simulink model "PMSM_Simulation"  (R2023a)
settings: Solver=ode23t  StartTime=0.0  StopTime=5  MaxStep=0.2  RelTol=1e-4  EnableMultiTasking=on
InitFcn:
  | p = 4;
  | Ld = 0.000425;
  | Lq = 0.00085;
  | psim = 0.119489;
  | Rs = 0.0485;
  | J = 0.00027;
  | Kpwm = 1;
  | Tsi = 0.0001;
  | h = 900;
  | 
  | L0 = (Ld+Lq)/2;
  | SMO_Kp = 100;
  | SMO_Coef =0.0001;
  | Ki_id = Ld*(h+1)/(4.5*Kpwm*(Tsi^2)*(h^2));
  | Kp_id = Ld*(h+1)/(4.5*Kpwm*Tsi*h);
  | 
  | wc =3000;
  | 
  | Ki_iq = Lq*(h+1)/(4.5*Kpwm*Tsi^2*h^2);
  | Kp_iq = Lq*(h+1)/(4.5*Kpwm*Tsi*h);
  | 
  | 
  | Kp_Spd = pi*J/(300*p*psim*Tsi)
  | Ki_Spd = pi*J/(6000*p*psim*Tsi^2)
  | 
  | DeadTime = 2e-6;
  | 
  | Udc = 650;
model workspace (MAT data in the model file):
  KfDeadCompen_CpPeriodTimesT_NULL : Simulink.Parameter (value not decoded)
  KfMDCC_InvParkCpPeriodTimesT_NULL : Simulink.Parameter (value not decoded)
values from neighbouring files (symbols this model uses):
  KfDeadCompen_SetDeltaTime_us = myPackage.Parameter    [DeadCompen.m]
  VbDeadComp_SwtUseIsttrDes_flg = myPackage.Parameter    [DeadCompen.m]
  VfDeadCompen_agIPredAdpr_C = myPackage.Parameter    [DeadCompen.m]
  VfDeadCompen_ISttrDdeThdSwt_A = myPackage.Parameter    [DeadCompen.m]
  VfDeadCompen_ISttrIgbtThdSwt_A = myPackage.Parameter    [DeadCompen.m]
  VfDeadCompen_rDdeISttrHi_R = myPackage.Parameter    [DeadCompen.m]
  VfDeadCompen_rDdeISttrLo_R = myPackage.Parameter    [DeadCompen.m]
  VfDeadCompen_rIgbtISttrHi_R = myPackage.Parameter    [DeadCompen.m]
  VfDeadCompen_rIgbtISttrLo_R = myPackage.Parameter    [DeadCompen.m]
  VfDeadCompen_uDdeISttrHi_V = myPackage.Parameter    [DeadCompen.m]
  VfDeadCompen_uDdeISttrLo_V = myPackage.Parameter    [DeadCompen.m]
  VfDeadCompen_uIgbtISttrHi_V = myPackage.Parameter    [DeadCompen.m]
  VfDeadCompen_uIgbtISttrLo_V = myPackage.Parameter    [DeadCompen.m]
symbols that are objects in the model workspace (value not decoded): KfDeadCompen_CpPeriodTimesT_NULL, KfMDCC_InvParkCpPeriodTimesT_NULL
undefined symbols (not defined in the file or in its folder): DiscIntNeverNeededParam, TableDeadTime_us, TableDeadTimeLookUpCur_A, VuDeadCompen_agIPredAdpr_C
libraries: simulink x23, mcbcontrolslib x11, mcbplantlib x1, spsCurrentMeasurementLib x1, spsDCVoltageSourceLib x1, spsMultimeterLib x1, spsPermanentMagnetSynchronousMachineLib x1, eePmsmCurrentController x1, spsThreePhaseVIMeasurementLib x1, spsUniversalBridgeLib x1, spspowerguiLib x1
(part 2 of 4)

== system PMSM_Simulation/Subsystem/Subsystem/Subsystem2/Subsystem ==
  U_Phase_Dyc : Inport
  V_Phase_Dyc : Inport  Port=2
  W_Phase_Dyc : Inport  Port=3
  iPhase_U : Inport  Port=4
  iPhase_V : Inport  Port=5
  iPhase_W : Inport  Port=6
  uDcLink : Inport  Port=7
  PwmFreq_Hz : Inport  Port=8
  Bus Creator : BusCreator  Inputs=4
  Bus Creator1 : BusCreator  Inputs=3
  DeadTimeDuty_Calc : Subsystem
  DeltaTimeOnOffDuty_Calc : Subsystem
  DutyErr_Calc : Subsystem  Commented=on  TreatAsAtomicUnit=on
  Tavon_Calc : Subsystem
  Bus_DutyCompensate : Outport
  wires:
  U_Phase_Dyc/1 -> Tavon_Calc/1(U_Phase_Dyc), Bus Creator1/1  "DutyPhaseU"
  V_Phase_Dyc/1 -> Bus Creator1/2, Tavon_Calc/2(V_Phase_Dyc)  "DutyPhaseV"
  W_Phase_Dyc/1 -> Bus Creator1/3, Tavon_Calc/3(W_Phase_Dyc)  "DutyPhaseW"
  iPhase_U/1 -> DeltaTimeOnOffDuty_Calc/1(iPhase_U), Tavon_Calc/4(iPhase_U)
  iPhase_V/1 -> DeltaTimeOnOffDuty_Calc/2(iPhase_V), Tavon_Calc/5(iPhase_V)
  iPhase_W/1 -> DeltaTimeOnOffDuty_Calc/3(iPhase_W), Tavon_Calc/6(iPhase_W)
  uDcLink/1 -> Tavon_Calc/7(uDcLink)
  PwmFreq_Hz/1 -> DeadTimeDuty_Calc/1(PwmFreq_Hz), DeltaTimeOnOffDuty_Calc/4(PwmFreq_Hz)
  Tavon_Calc/1(Bus_DutyAvon) -> Bus Creator/2  "Bus_DutyAvon"
  DeltaTimeOnOffDuty_Calc/1(Bus_DeltaTimeOnOffDuty) -> Bus Creator/3  "Bus_DeltaTimeOnOffDuty"
  DeadTimeDuty_Calc/1(DeadTimeDuty_NULL) -> Bus Creator/4  "DeadTimeDuty_NULL"
  Bus Creator/1 -> Bus_DutyCompensate/1  "Bus_DutyCompensate"
  Bus Creator1/1 -> Bus Creator/1  "SVM_DutyPhase"

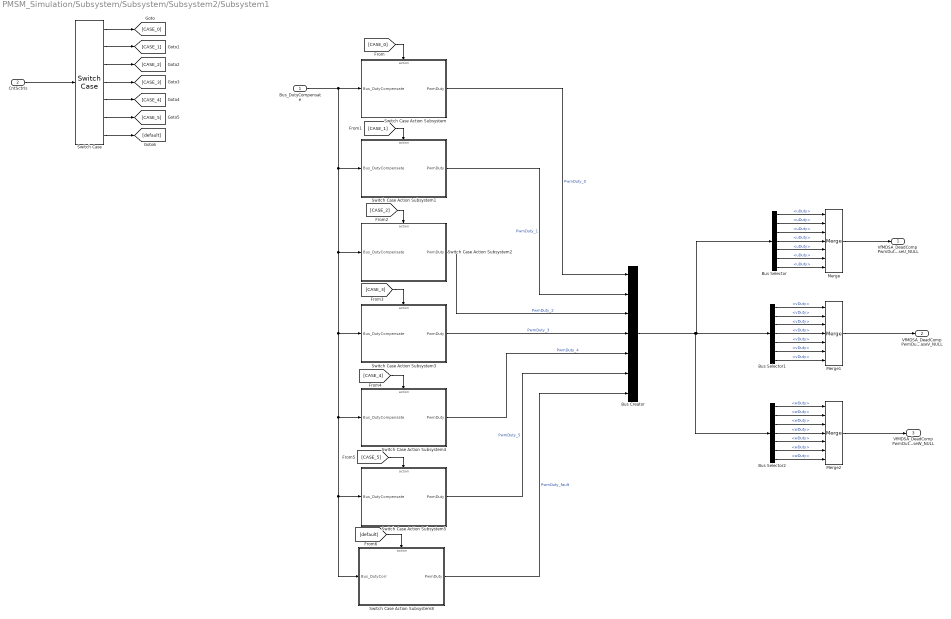
== system PMSM_Simulation/Subsystem/Subsystem/Subsystem2/Subsystem1 ==
  Bus_DutyCompensate : Inport
  CntSctrIs : Inport  Port=2
  Bus Creator : BusCreator  Inputs=7
  Bus Selector : BusSelector  OutputSignals=PwmDuty_0.uDuty,PwmDuty_1.uDuty,PwmDuty_2.uDuty,PwmDuty_3.uDuty,PwmDuty_4.uDuty,PwmDuty_5.uDuty,PwmDuty_fault.uDuty
  Bus Selector1 : BusSelector  OutputSignals=PwmDuty_1.vDuty,PwmDuty_0.vDuty,PwmDuty_2.vDuty,PwmDuty_3.vDuty,PwmDuty_4.vDuty,PwmDuty_5.vDuty,PwmDuty_fault.vDuty
  Bus Selector2 : BusSelector  OutputSignals=PwmDuty_0.wDuty,PwmDuty_1.wDuty,PwmDuty_2.wDuty,PwmDuty_3.wDuty,PwmDuty_4.wDuty,PwmDuty_5.wDuty,PwmDuty_fault.wDuty
  Merge : Merge  Inputs=7
  Merge1 : Merge  Inputs=7
  Merge2 : Merge  Inputs=7
  Switch Case : SwitchCase  CaseConditions={0,1,2,3,4,5}
  Switch Case Action Subsystem : Subsystem  TreatAsAtomicUnit=on
  Switch Case Action Subsystem1 : Subsystem  TreatAsAtomicUnit=on
  Switch Case Action Subsystem2 : Subsystem  TreatAsAtomicUnit=on
  Switch Case Action Subsystem3 : Subsystem  TreatAsAtomicUnit=on
  Switch Case Action Subsystem4 : Subsystem  TreatAsAtomicUnit=on
  Switch Case Action Subsystem5 : Subsystem  TreatAsAtomicUnit=on
  Switch Case Action Subsystem8 : Subsystem  TreatAsAtomicUnit=on
  VfMDSA_DeadCompPwmDutyCyclePhaseU_NULL : Outport
  VfMDSA_DeadCompPwmDutyCyclePhaseV_NULL : Outport  Port=2
  VfMDSA_DeadCompPwmDutyCyclePhaseW_NULL : Outport  Port=3
  wires:
  CntSctrIs/1 -> Switch Case/1
  Switch Case/1 -> [CASE_0]
  Switch Case/2 -> [CASE_1]
  Switch Case/3 -> [CASE_2]
  Switch Case/4 -> [CASE_3]
  Switch Case/5 -> [CASE_4]
  Switch Case/7 -> [default]
  [CASE_0] -> Switch Case Action Subsystem/Action
  [CASE_1] -> Switch Case Action Subsystem1/Action
  [CASE_2] -> Switch Case Action Subsystem2/Action
  [CASE_3] -> Switch Case Action Subsystem3/Action
  [CASE_4] -> Switch Case Action Subsystem4/Action
  [CASE_5] -> Switch Case Action Subsystem5/Action
  [default] -> Switch Case Action Subsystem8/Action
  Switch Case/6 -> [CASE_5]
  Merge/1 -> VfMDSA_DeadCompPwmDutyCyclePhaseU_NULL/1
  Switch Case Action Subsystem/1(PwmDuty) -> Bus Creator/1  "PwmDuty_0"
  Switch Case Action Subsystem1/1(PwmDuty) -> Bus Creator/2  "PwmDuty_1"
  Switch Case Action Subsystem2/1(PwmDuty) -> Bus Creator/3  "PwmDuty_2"
  Switch Case Action Subsystem3/1(PwmDuty) -> Bus Creator/4  "PwmDuty_3"
  Switch Case Action Subsystem4/1(PwmDuty) -> Bus Creator/5  "PwmDuty_4"
  Switch Case Action Subsystem5/1(PwmDuty) -> Bus Creator/6  "PwmDuty_5"
  Switch Case Action Subsystem8/1(PwmDuty) -> Bus Creator/7  "PwmDuty_fault"
  Merge1/1 -> VfMDSA_DeadCompPwmDutyCyclePhaseV_NULL/1
  Merge2/1 -> VfMDSA_DeadCompPwmDutyCyclePhaseW_NULL/1
  Bus Creator/1 -> Bus Selector2/1, Bus Selector1/1, Bus Selector/1
  Bus Selector/1 -> Merge/1  "<uDuty>"
  Bus Selector/2 -> Merge/2  "<uDuty>"
  Bus Selector/3 -> Merge/3  "<uDuty>"
  Bus Selector/4 -> Merge/4  "<uDuty>"
  Bus Selector/5 -> Merge/5  "<uDuty>"
  Bus Selector/6 -> Merge/6  "<uDuty>"
  Bus Selector/7 -> Merge/7  "<uDuty>"
  Bus Selector1/1 -> Merge1/1  "<vDuty>"
  Bus Selector1/2 -> Merge1/2  "<vDuty>"
  Bus Selector1/3 -> Merge1/3  "<vDuty>"
  Bus Selector1/4 -> Merge1/4  "<vDuty>"
  Bus Selector1/5 -> Merge1/5  "<vDuty>"
  Bus Selector1/6 -> Merge1/6  "<vDuty>"
  Bus Selector1/7 -> Merge1/7  "<vDuty>"
  Bus Selector2/1 -> Merge2/1  "<wDuty>"
  Bus Selector2/2 -> Merge2/2  "<wDuty>"
  Bus Selector2/3 -> Merge2/3  "<wDuty>"
  Bus Selector2/4 -> Merge2/4  "<wDuty>"
  Bus Selector2/5 -> Merge2/5  "<wDuty>"
  Bus Selector2/6 -> Merge2/6  "<wDuty>"
  Bus Selector2/7 -> Merge2/7  "<wDuty>"
  Bus_DutyCompensate/1 -> Switch Case Action Subsystem1/1(Bus_DutyCompensate), Switch Case Action Subsystem2/1(Bus_DutyCompensate), Switch Case Action Subsystem3/1(Bus_DutyCompensate), Switch Case Action Subsystem4/1(Bus_DutyCompensate), Switch Case Action Subsystem5/1(Bus_DutyCompensate), Switch Case Action Subsystem8/1("Bus_DutyCorr "), Switch Case Action Subsystem/1(Bus_DutyCompensate)

== system PMSM_Simulation/Subsystem/Subsystem/Subsystem2/Subsystem2 ==
  IsdDes_A : Inport
  IsqDes_A : Inport  Port=2
  IsdFb_A : Inport  Port=3
  IsqFb_A : Inport  Port=4
  FrqRtrEl_Hz : Inport  Port=5
  agPreRtrEl : Inport  Port=6
  PwmFreq_Hz : Inport  Port=7
  Gain : Gain  Gain=6*pi
  Inverse Clarke Transform : mcbcontrolslib/Inverse Clarke Transform
  Inverse Park Transform : mcbcontrolslib/Inverse Park Transform  AxisAlignment=D-axis
  Sine-Cosine Lookup : mcbcontrolslib/Sine-Cosine Lookup  AngleInput=Radians  N_points=4095
  Subsystem1 : Subsystem
  Subsystem3 : Subsystem
  iaPre : Outport
  ibPre : Outport  Port=2
  icPre : Outport  Port=3
  CntSctrIs : Outport  Port=4
  wires:
  Inverse Park Transform/1 -> Inverse Clarke Transform/1
  Subsystem1/2(Isq_A) -> Subsystem3/5(Isq_A), Inverse Park Transform/2
  IsdDes_A/1 -> Subsystem1/1(IsdDes_A)
  Subsystem1/1(Isd_A) -> Inverse Park Transform/1, Subsystem3/4(Isd_A)
  Sine-Cosine Lookup/2 -> Inverse Park Transform/4
  Inverse Clarke Transform/2 -> ibPre/1
  Sine-Cosine Lookup/1 -> Inverse Park Transform/3
  IsqFb_A/1 -> Subsystem1/4(IsqFb_A)
  Inverse Clarke Transform/3 -> icPre/1
  Inverse Park Transform/2 -> Inverse Clarke Transform/2
  IsdFb_A/1 -> Subsystem1/3(IsdFb_A)
  FrqRtrEl_Hz/1 -> Gain/1
  IsqDes_A/1 -> Subsystem1/2(IsqDes_A)
  agPreRtrEl/1 -> Subsystem3/2(eMtrPos_NULL)
  Inverse Clarke Transform/1 -> iaPre/1
  PwmFreq_Hz/1 -> Subsystem3/3(VfPwmFreq_Hz)
  Gain/1 -> Subsystem3/1(eMtrSpd_rads)
  Subsystem3/2(Select_N) -> CntSctrIs/1
  Subsystem3/1(PreMtrPos) -> Sine-Cosine Lookup/1

== system PMSM_Simulation/Subsystem/Subsystem/Subsystem4/Subsystem1 ==
  In1 : Inport
  In2 : Inport  Port=2
  Add : Sum  Inputs=+-
  Constant : Constant  OutDataTypeStr=single
  Gain : Gain  Gain=2
  Product : Product
  Subsystem : Subsystem
  Out1 : Outport
  wires:
  In2/1 -> Gain/1
  Gain/1 -> Add/1
  Constant/1 -> Add/2
  Add/1 -> Product/2
  Product/1 -> Out1/1
  In1/1 -> Subsystem/1(In1)
  Subsystem/1(Out1) -> Product/1

== system PMSM_Simulation/Subsystem/Subsystem/Subsystem4/Subsystem2 ==
  In1 : Inport
  In2 : Inport  Port=2
  Add : Sum  Inputs=+-
  Constant : Constant  OutDataTypeStr=single
  Gain : Gain  Gain=2
  Product : Product
  Subsystem : Subsystem
  Out1 : Outport
  wires:
  In2/1 -> Gain/1
  Gain/1 -> Add/1
  Constant/1 -> Add/2
  Add/1 -> Product/2
  Product/1 -> Out1/1
  In1/1 -> Subsystem/1(In1)
  Subsystem/1(Out1) -> Product/1

== system PMSM_Simulation/Subsystem/Subsystem/Subsystem4/Subsystem3 ==
  In1 : Inport
  In2 : Inport  Port=2
  Add : Sum  Inputs=+-
  Constant : Constant  OutDataTypeStr=single
  Gain : Gain  Gain=2
  Product : Product
  Subsystem : Subsystem
  Out1 : Outport
  wires:
  In2/1 -> Gain/1
  Gain/1 -> Add/1
  Constant/1 -> Add/2
  Add/1 -> Product/2
  Product/1 -> Out1/1
  In1/1 -> Subsystem/1(In1)
  Subsystem/1(Out1) -> Product/1

== system PMSM_Simulation/Subsystem/Subsystem/DeadComp_Sys/Subsystem/DeadTimeDuty_Calc ==
  PwmFreq_Hz : Inport
  Constant : Constant  Value=KfDeadCompen_SetDeltaTime_us  OutDataTypeStr=single
  Constant1 : Constant  Value=1e6  OutDataTypeStr=single
  Divide2 : Product  Inputs=**/
  DeadTimeDuty_NULL : Outport
  wires:
  Divide2/1 -> DeadTimeDuty_NULL/1  "DeadTimeDuty_NULL"
  Constant/1 -> Divide2/1
  Constant1/1 -> Divide2/3
  PwmFreq_Hz/1 -> Divide2/2

== system PMSM_Simulation/Subsystem/Subsystem/DeadComp_Sys/Subsystem/DeltaTimeOnOffDuty_Calc ==
  iPhase_U : Inport
  iPhase_V : Inport  Port=2
  iPhase_W : Inport  Port=3
  PwmFreq_Hz : Inport  Port=4
  1-D Lookup Table1 : Lookup_n-D  Priority=48  NumberOfTableDimensions=1  BreakpointsForDimension1=TableDeadTimeLookUpCur_A  Table=TableDeadTime_us  InternalRulePriority=Speed  RndMeth=Simplest
  1-D Lookup Table2 : Lookup_n-D  Priority=48  NumberOfTableDimensions=1  BreakpointsForDimension1=TableDeadTimeLookUpCur_A  Table=TableDeadTime_us  InternalRulePriority=Speed  RndMeth=Simplest
  1-D Lookup Table3 : Lookup_n-D  Priority=48  NumberOfTableDimensions=1  BreakpointsForDimension1=TableDeadTimeLookUpCur_A  Table=TableDeadTime_us  InternalRulePriority=Speed  RndMeth=Simplest
  Abs : Abs  Priority=39  SaturateOnIntegerOverflow=off
  Abs1 : Abs  Priority=47  SaturateOnIntegerOverflow=off
  Abs2 : Abs  Priority=51  SaturateOnIntegerOverflow=off
  Bus Creator : BusCreator  Inputs=3
  Constant : Constant  Value=1e6  OutDataTypeStr=single
  Divide : Product  Inputs=**/
  Divide1 : Product  Inputs=**/
  Divide2 : Product  Inputs=**/
  Bus_DeltaTimeOnOffDuty : Outport
  wires:
  1-D Lookup Table1/1 -> Divide/1
  1-D Lookup Table3/1 -> Divide2/1
  PwmFreq_Hz/1 -> Divide/2, Divide1/2, Divide2/2
  iPhase_U/1 -> Abs/1
  1-D Lookup Table2/1 -> Divide1/1
  Bus Creator/1 -> Bus_DeltaTimeOnOffDuty/1
  Abs2/1 -> 1-D Lookup Table3/1  "iPhaseAbs"
  iPhase_V/1 -> Abs1/1
  Constant/1 -> Divide/3, Divide1/3, Divide2/3
  Abs1/1 -> 1-D Lookup Table2/1  "iPhaseAbs"
  Abs/1 -> 1-D Lookup Table1/1  "iPhaseAbs"
  Divide1/1 -> Bus Creator/2  "DeltaTimeOnOffV_NULL"
  Divide/1 -> Bus Creator/1  "DeltaTimeOnOffU_NULL"
  Divide2/1 -> Bus Creator/3  "DeltaTimeOnOffW_NULL"
  iPhase_W/1 -> Abs2/1

== system PMSM_Simulation/Subsystem/Subsystem/DeadComp_Sys/Subsystem/Tavon_Calc ==
  U_Phase_Dyc : Inport
  V_Phase_Dyc : Inport  Port=2
  W_Phase_Dyc : Inport  Port=3
  iPhase_U : Inport  Port=4
  iPhase_V : Inport  Port=5
  iPhase_W : Inport  Port=6
  uDcLink : Inport  Port=7
  Bus Creator : BusCreator  Inputs=3
  ia : Subsystem
  ia1 : Subsystem
  ia2 : Subsystem
  Bus_DutyAvon : Outport
  wires:
  V_Phase_Dyc/1 -> ia1/2(Phase_Dyc)
  ia1/1("Duty_Avon ") -> Bus Creator/2  "DutyAvon_V"
  U_Phase_Dyc/1 -> ia/2(Phase_Dyc)
  uDcLink/1 -> ia2/3(uDcLink), ia1/3(uDcLink), ia/3(uDcLink)
  iPhase_V/1 -> ia1/1(iPhase)
  ia2/1("Duty_Avon ") -> Bus Creator/3  "DutyAvon_W"
  iPhase_W/1 -> ia2/1(iPhase)
  W_Phase_Dyc/1 -> ia2/2(Phase_Dyc)
  Bus Creator/1 -> Bus_DutyAvon/1  "DutyAvon"
  iPhase_U/1 -> ia/1(iPhase)
  ia/1("Duty_Avon ") -> Bus Creator/1  "DutyAvon_U"

== system PMSM_Simulation/Subsystem/Subsystem/DeadComp_Sys/Subsystem1/Switch Case Action Subsystem ==
  Bus_DutyCompensate : Inport
  Action Port : ActionPort
  Add : Sum  Inputs=++-
  Add1 : Sum  Inputs=+-+
  Add2 : Sum  Inputs=+-+
  Bus Creator : BusCreator  Inputs=3
  Bus Selector : BusSelector  OutputSignals=Bus_DutyAvon.DutyAvon_U,DeadTimeDuty_NULL,Bus_DeltaTimeOnOffDuty.DeltaTimeOnOffU_NULL
  Bus Selector1 : BusSelector  OutputSignals=Bus_DutyAvon.DutyAvon_V,DeadTimeDuty_NULL,Bus_DeltaTimeOnOffDuty.DeltaTimeOnOffV_NULL
  Bus Selector2 : BusSelector  OutputSignals=Bus_DutyAvon.DutyAvon_W,DeadTimeDuty_NULL,Bus_DeltaTimeOnOffDuty.DeltaTimeOnOffW_NULL
  PwmDuty : Outport
  wires:
  Add/1 -> Bus Creator/1  "uDuty"
  Add1/1 -> Bus Creator/2  "vDuty"
  Add2/1 -> Bus Creator/3  "wDuty"
  Bus Creator/1 -> PwmDuty/1
  Bus_DutyCompensate/1 -> Bus Selector/1, Bus Selector2/1, Bus Selector1/1
  Bus Selector/1 -> Add/1  "<DutyAvon_U>"
  Bus Selector/3 -> Add/3  "<DeltaTimeOnOffU_NULL>"
  Bus Selector1/2 -> Add1/2  "<DeadTimeDuty_NULL>"
  Bus Selector1/1 -> Add1/1  "<DutyAvon_V>"
  Bus Selector2/1 -> Add2/1  "<DutyAvon_W>"
  Bus Selector2/2 -> Add2/2  "<DeadTimeDuty_NULL>"
  Bus Selector/2 -> Add/2  "<DeadTimeDuty_NULL>"
  Bus Selector1/3 -> Add1/3  "<DeltaTimeOnOffV_NULL>"
  Bus Selector2/3 -> Add2/3  "<DeltaTimeOnOffW_NULL>"

== system PMSM_Simulation/Subsystem/Subsystem/DeadComp_Sys/Subsystem1/Switch Case Action Subsystem1 ==
  Bus_DutyCompensate : Inport
  Action Port : ActionPort
  Add : Sum  Inputs=++-
  Add1 : Sum  Inputs=++-
  Add2 : Sum  Inputs=+-+
  Bus Creator : BusCreator  Inputs=3
  Bus Selector : BusSelector  OutputSignals=Bus_DutyAvon.DutyAvon_U,DeadTimeDuty_NULL,Bus_DeltaTimeOnOffDuty.DeltaTimeOnOffU_NULL
  Bus Selector1 : BusSelector  OutputSignals=Bus_DutyAvon.DutyAvon_V,DeadTimeDuty_NULL,Bus_DeltaTimeOnOffDuty.DeltaTimeOnOffV_NULL
  Bus Selector2 : BusSelector  OutputSignals=Bus_DutyAvon.DutyAvon_W,DeadTimeDuty_NULL,Bus_DeltaTimeOnOffDuty.DeltaTimeOnOffW_NULL
  PwmDuty : Outport
  wires:
  Add/1 -> Bus Creator/1  "uDuty"
  Add1/1 -> Bus Creator/2  "vDuty"
  Add2/1 -> Bus Creator/3  "wDuty"
  Bus Creator/1 -> PwmDuty/1
  Bus_DutyCompensate/1 -> Bus Selector/1, Bus Selector2/1, Bus Selector1/1
  Bus Selector/1 -> Add/1  "<DutyAvon_U>"
  Bus Selector/3 -> Add/3  "<DeltaTimeOnOffU_NULL>"
  Bus Selector1/2 -> Add1/2  "<DeadTimeDuty_NULL>"
  Bus Selector1/1 -> Add1/1  "<DutyAvon_V>"
  Bus Selector2/1 -> Add2/1  "<DutyAvon_W>"
  Bus Selector2/2 -> Add2/2  "<DeadTimeDuty_NULL>"
  Bus Selector/2 -> Add/2  "<DeadTimeDuty_NULL>"
  Bus Selector1/3 -> Add1/3  "<DeltaTimeOnOffV_NULL>"
  Bus Selector2/3 -> Add2/3  "<DeltaTimeOnOffW_NULL>"

== system PMSM_Simulation/Subsystem/Subsystem/DeadComp_Sys/Subsystem1/Switch Case Action Subsystem2 ==
  Bus_DutyCompensate : Inport
  Action Port : ActionPort
  Add : Sum  Inputs=+-+
  Add1 : Sum  Inputs=++-
  Add2 : Sum  Inputs=+-+
  Bus Creator : BusCreator  Inputs=3
  Bus Selector : BusSelector  OutputSignals=Bus_DutyAvon.DutyAvon_U,DeadTimeDuty_NULL,Bus_DeltaTimeOnOffDuty.DeltaTimeOnOffU_NULL
  Bus Selector1 : BusSelector  OutputSignals=Bus_DutyAvon.DutyAvon_V,DeadTimeDuty_NULL,Bus_DeltaTimeOnOffDuty.DeltaTimeOnOffV_NULL
  Bus Selector2 : BusSelector  OutputSignals=Bus_DutyAvon.DutyAvon_W,DeadTimeDuty_NULL,Bus_DeltaTimeOnOffDuty.DeltaTimeOnOffW_NULL
  PwmDuty : Outport
  wires:
  Add/1 -> Bus Creator/1  "uDuty"
  Add1/1 -> Bus Creator/2  "vDuty"
  Add2/1 -> Bus Creator/3  "wDuty"
  Bus Creator/1 -> PwmDuty/1
  Bus_DutyCompensate/1 -> Bus Selector/1, Bus Selector2/1, Bus Selector1/1
  Bus Selector/1 -> Add/1  "<DutyAvon_U>"
  Bus Selector/3 -> Add/3  "<DeltaTimeOnOffU_NULL>"
  Bus Selector1/2 -> Add1/2  "<DeadTimeDuty_NULL>"
  Bus Selector1/1 -> Add1/1  "<DutyAvon_V>"
  Bus Selector2/1 -> Add2/1  "<DutyAvon_W>"
  Bus Selector2/2 -> Add2/2  "<DeadTimeDuty_NULL>"
  Bus Selector/2 -> Add/2  "<DeadTimeDuty_NULL>"
  Bus Selector1/3 -> Add1/3  "<DeltaTimeOnOffV_NULL>"
  Bus Selector2/3 -> Add2/3  "<DeltaTimeOnOffW_NULL>"

== system PMSM_Simulation/Subsystem/Subsystem/DeadComp_Sys/Subsystem1/Switch Case Action Subsystem3 ==
  Bus_DutyCompensate : Inport
  Action Port : ActionPort
  Add : Sum  Inputs=+-+
  Add1 : Sum  Inputs=++-
  Add2 : Sum  Inputs=++-
  Bus Creator : BusCreator  Inputs=3
  Bus Selector : BusSelector  OutputSignals=Bus_DutyAvon.DutyAvon_U,DeadTimeDuty_NULL,Bus_DeltaTimeOnOffDuty.DeltaTimeOnOffU_NULL
  Bus Selector1 : BusSelector  OutputSignals=Bus_DutyAvon.DutyAvon_V,DeadTimeDuty_NULL,Bus_DeltaTimeOnOffDuty.DeltaTimeOnOffV_NULL
  Bus Selector2 : BusSelector  OutputSignals=Bus_DutyAvon.DutyAvon_W,DeadTimeDuty_NULL,Bus_DeltaTimeOnOffDuty.DeltaTimeOnOffW_NULL
  PwmDuty : Outport
  wires:
  Add/1 -> Bus Creator/1  "uDuty"
  Add1/1 -> Bus Creator/2  "vDuty"
  Add2/1 -> Bus Creator/3  "wDuty"
  Bus Creator/1 -> PwmDuty/1
  Bus_DutyCompensate/1 -> Bus Selector/1, Bus Selector2/1, Bus Selector1/1
  Bus Selector/1 -> Add/1  "<DutyAvon_U>"
  Bus Selector/3 -> Add/3  "<DeltaTimeOnOffU_NULL>"
  Bus Selector1/2 -> Add1/2  "<DeadTimeDuty_NULL>"
  Bus Selector1/1 -> Add1/1  "<DutyAvon_V>"
  Bus Selector2/1 -> Add2/1  "<DutyAvon_W>"
  Bus Selector2/2 -> Add2/2  "<DeadTimeDuty_NULL>"
  Bus Selector/2 -> Add/2  "<DeadTimeDuty_NULL>"
  Bus Selector1/3 -> Add1/3  "<DeltaTimeOnOffV_NULL>"
  Bus Selector2/3 -> Add2/3  "<DeltaTimeOnOffW_NULL>"

== system PMSM_Simulation/Subsystem/Subsystem/DeadComp_Sys/Subsystem1/Switch Case Action Subsystem4 ==
  Bus_DutyCompensate : Inport
  Action Port : ActionPort
  Add : Sum  Inputs=+-+
  Add1 : Sum  Inputs=+-+
  Add2 : Sum  Inputs=++-
  Bus Creator : BusCreator  Inputs=3
  Bus Selector : BusSelector  OutputSignals=Bus_DutyAvon.DutyAvon_U,DeadTimeDuty_NULL,Bus_DeltaTimeOnOffDuty.DeltaTimeOnOffU_NULL
  Bus Selector1 : BusSelector  OutputSignals=Bus_DutyAvon.DutyAvon_V,DeadTimeDuty_NULL,Bus_DeltaTimeOnOffDuty.DeltaTimeOnOffV_NULL
  Bus Selector2 : BusSelector  OutputSignals=Bus_DutyAvon.DutyAvon_W,DeadTimeDuty_NULL,Bus_DeltaTimeOnOffDuty.DeltaTimeOnOffW_NULL
  PwmDuty : Outport
  wires:
  Add/1 -> Bus Creator/1  "uDuty"
  Add1/1 -> Bus Creator/2  "vDuty"
  Add2/1 -> Bus Creator/3  "wDuty"
  Bus Creator/1 -> PwmDuty/1
  Bus_DutyCompensate/1 -> Bus Selector/1, Bus Selector2/1, Bus Selector1/1
  Bus Selector/1 -> Add/1  "<DutyAvon_U>"
  Bus Selector/3 -> Add/3  "<DeltaTimeOnOffU_NULL>"
  Bus Selector1/2 -> Add1/2  "<DeadTimeDuty_NULL>"
  Bus Selector1/1 -> Add1/1  "<DutyAvon_V>"
  Bus Selector2/1 -> Add2/1  "<DutyAvon_W>"
  Bus Selector2/2 -> Add2/2  "<DeadTimeDuty_NULL>"
  Bus Selector/2 -> Add/2  "<DeadTimeDuty_NULL>"
  Bus Selector1/3 -> Add1/3  "<DeltaTimeOnOffV_NULL>"
  Bus Selector2/3 -> Add2/3  "<DeltaTimeOnOffW_NULL>"

== system PMSM_Simulation/Subsystem/Subsystem/DeadComp_Sys/Subsystem1/Switch Case Action Subsystem5 ==
  Bus_DutyCompensate : Inport
  Action Port : ActionPort
  Add : Sum  Inputs=++-
  Add1 : Sum  Inputs=+-+
  Add2 : Sum  Inputs=++-
  Bus Creator : BusCreator  Inputs=3
  Bus Selector : BusSelector  OutputSignals=Bus_DutyAvon.DutyAvon_U,DeadTimeDuty_NULL,Bus_DeltaTimeOnOffDuty.DeltaTimeOnOffU_NULL
  Bus Selector1 : BusSelector  OutputSignals=Bus_DutyAvon.DutyAvon_V,DeadTimeDuty_NULL,Bus_DeltaTimeOnOffDuty.DeltaTimeOnOffV_NULL
  Bus Selector2 : BusSelector  OutputSignals=Bus_DutyAvon.DutyAvon_W,DeadTimeDuty_NULL,Bus_DeltaTimeOnOffDuty.DeltaTimeOnOffW_NULL
  PwmDuty : Outport
  wires:
  Add/1 -> Bus Creator/1  "uDuty"
  Add1/1 -> Bus Creator/2  "vDuty"
  Add2/1 -> Bus Creator/3  "wDuty"
  Bus Creator/1 -> PwmDuty/1
  Bus_DutyCompensate/1 -> Bus Selector/1, Bus Selector2/1, Bus Selector1/1
  Bus Selector/1 -> Add/1  "<DutyAvon_U>"
  Bus Selector/3 -> Add/3  "<DeltaTimeOnOffU_NULL>"
  Bus Selector1/2 -> Add1/2  "<DeadTimeDuty_NULL>"
  Bus Selector1/1 -> Add1/1  "<DutyAvon_V>"
  Bus Selector2/1 -> Add2/1  "<DutyAvon_W>"
  Bus Selector2/2 -> Add2/2  "<DeadTimeDuty_NULL>"
  Bus Selector/2 -> Add/2  "<DeadTimeDuty_NULL>"
  Bus Selector1/3 -> Add1/3  "<DeltaTimeOnOffV_NULL>"
  Bus Selector2/3 -> Add2/3  "<DeltaTimeOnOffW_NULL>"

== system PMSM_Simulation/Subsystem/Subsystem/DeadComp_Sys/Subsystem1/Switch Case Action Subsystem8 ==
  "Bus_DutyCorr " : Inport
  Action Port : ActionPort
  Bus Creator : BusCreator  Inputs=3
  Bus Selector : BusSelector  OutputSignals=SVM_DutyPhase.DutyPhaseU,SVM_DutyPhase.DutyPhaseV,SVM_DutyPhase.DutyPhaseW
  Signal Copy : SignalConversion  OverrideOpt=off
  Signal Copy1 : SignalConversion  OverrideOpt=off
  Signal Copy2 : SignalConversion  OverrideOpt=off
  PwmDuty : Outport
  wires:
  "Bus_DutyCorr "/1 -> Bus Selector/1
  Bus Selector/1 -> Signal Copy/1  "<DutyPhaseU>"
  Signal Copy1/1 -> Bus Creator/2  "vDuty"
  Bus Creator/1 -> PwmDuty/1
  Signal Copy2/1 -> Bus Creator/3  "wDuty"
  Signal Copy/1 -> Bus Creator/1  "uDuty"
  Bus Selector/2 -> Signal Copy1/1  "<DutyPhaseV>"
  Bus Selector/3 -> Signal Copy2/1  "<DutyPhaseW>"

== system PMSM_Simulation/Subsystem/Subsystem/DeadComp_Sys/Subsystem2/Subsystem1 ==
  IsdDes_A : Inport
  IsqDes_A : Inport  Port=2
  IsdFb_A : Inport  Port=3
  IsqFb_A : Inport  Port=4
  Bus Creator : BusCreator  Inputs=2
  Bus Creator1 : BusCreator  Inputs=2
  Bus Selector : BusSelector  OutputSignals=Isd_A,Isq_A
  Constant : Constant  Value=VbDeadComp_SwtUseIsttrDes_flg
  Switch : Switch  Criteria=u2 ~= 0  SaturateOnIntegerOverflow=off  InputSameDT=off
  Isd_A : Outport
  Isq_A : Outport  Port=2
  wires:
  Bus Creator1/1 -> Switch/3
  IsqDes_A/1 -> Bus Creator/2  "Isq_A"
  Bus Creator/1 -> Switch/1
  IsqFb_A/1 -> Bus Creator1/2  "Isq_A"
  IsdFb_A/1 -> Bus Creator1/1  "Isd_A"
  Constant/1 -> Switch/2
  IsdDes_A/1 -> Bus Creator/1  "Isd_A"
  Switch/1 -> Bus Selector/1
  Bus Selector/1 -> Isd_A/1  "<Isd_A>"
  Bus Selector/2 -> Isq_A/1  "<Isq_A>"

== system PMSM_Simulation/Subsystem/Subsystem/DeadComp_Sys/Subsystem2/Subsystem3 ==
  eMtrSpd_rads : Inport
  eMtrPos_NULL : Inport  Port=2
  VfPwmFreq_Hz : Inport  Port=3
  Isd_A : Inport  Port=4
  Isq_A : Inport  Port=5
  Add : Sum  Inputs=+++
  Constant2 : Constant  Value=2*pi  OutDataTypeStr=single
  Constant3 : Constant  Value=pi/6  OutDataTypeStr=single
  Constant4 : Constant  Value=pi/3  OutDataTypeStr=single
  Data Type Conversion : DataTypeConversion  OutDataTypeStr=uint8  SaturateOnIntegerOverflow=off  RndMeth=Floor
  Divide : Product  Inputs=*/
  Mod : Math  Operator=mod
  Subsystem1 : Subsystem
  Subsystem2 : Subsystem
  PreMtrPos : Outport
  Select_N : Outport  Port=2
  wires:
  Constant3/1 -> Add/3
  Mod/1 -> Divide/1
  Subsystem2/1(PreMtrPos) -> PreMtrPos/1, Add/1
  Constant2/1 -> Mod/2
  eMtrPos_NULL/1 -> Subsystem2/2(eMtrPos_NULL)
  Add/1 -> Mod/1
  Subsystem1/1(agIsE) -> Add/2
  Divide/1 -> Data Type Conversion/1
  Constant4/1 -> Divide/2
  Data Type Conversion/1 -> Select_N/1
  Isq_A/1 -> Subsystem1/2(Isq_A)
  Isd_A/1 -> Subsystem1/1(Isd_A)
  VfPwmFreq_Hz/1 -> Subsystem2/3(VfPwmFreq_Hz)
  eMtrSpd_rads/1 -> Subsystem2/1(eMtrSpd_rads)

== system PMSM_Simulation/Subsystem/Subsystem/SMO/Subsystem/Subsystem ==
  In1 : Inport
  Add1 : Sum
  Add2 : Sum  Inputs=-+
  Constant : Constant  Value=SMO_Coef
  Constant1 : Constant
  Delay : Delay  DelayLength=1
  Product1 : Product
  Product2 : Product
  Ealpha : Outport
  wires:
  Product1/1 -> Add1/1
  Constant/1 -> Add2/1, Product1/2
  Add1/1 -> Ealpha/1, Delay/1
  Constant1/1 -> Add2/2
  In1/1 -> Product1/1
  Product2/1 -> Add1/2
  Add2/1 -> Product2/1
  Delay/1 -> Product2/2

== system PMSM_Simulation/Subsystem/Subsystem/SMO/Subsystem1/Subsystem ==
  In1 : Inport
  Add1 : Sum
  Add2 : Sum  Inputs=-+
  Constant : Constant  Value=SMO_Coef
  Constant1 : Constant
  Delay : Delay  DelayLength=1
  Product1 : Product
  Product2 : Product
  Ealpha : Outport
  wires:
  Product1/1 -> Add1/1
  Constant/1 -> Add2/1, Product1/2
  Add1/1 -> Ealpha/1, Delay/1
  Constant1/1 -> Add2/2
  In1/1 -> Product1/1
  Product2/1 -> Add1/2
  Add2/1 -> Product2/1
  Delay/1 -> Product2/2

== system PMSM_Simulation/Subsystem/Subsystem/SMO1/Ealpha_calc/Subsystem ==
  In1 : Inport
  Add1 : Sum
  Add2 : Sum  Inputs=-+
  Constant : Constant  Value=SMO_Coef
  Constant1 : Constant
  Delay : Delay  DelayLength=1
  Product1 : Product
  Product2 : Product
  Ealpha : Outport
  wires:
  Product1/1 -> Add1/1
  Constant/1 -> Add2/1, Product1/2
  Add1/1 -> Ealpha/1, Delay/1
  Constant1/1 -> Add2/2
  In1/1 -> Product1/1
  Product2/1 -> Add1/2
  Add2/1 -> Product2/1
  Delay/1 -> Product2/2

== system PMSM_Simulation/Subsystem/Subsystem/SMO1/Ebeta_Calc/Subsystem ==
  In1 : Inport
  Add1 : Sum
  Add2 : Sum  Inputs=-+
  Constant : Constant  Value=SMO_Coef
  Constant1 : Constant
  Delay : Delay  DelayLength=1
  Product1 : Product
  Product2 : Product
  Ealpha : Outport
  wires:
  Product1/1 -> Add1/1
  Constant/1 -> Add2/1, Product1/2
  Add1/1 -> Ealpha/1, Delay/1
  Constant1/1 -> Add2/2
  In1/1 -> Product1/1
  Product2/1 -> Add1/2
  Add2/1 -> Product2/1
  Delay/1 -> Product2/2

== system PMSM_Simulation/Subsystem/Subsystem/SVM_PU/N_Sector_calc/N_calc ==
  Uref1 : Inport
  Uref2 : Inport  Port=2
  Uref3 : Inport  Port=3
  Add : Sum  Inputs=+++
  ConstanT1 : Constant  Value=0  OutDataTypeStr=single
  Constant : Constant  OutDataTypeStr=single
  Gain : Gain
  Gain1 : Gain  Gain=2
  Gain2 : Gain  Gain=4
  Switch : Switch  Criteria=u2 > Threshold  SaturateOnIntegerOverflow=off  InputSameDT=off
  Switch1 : Switch  Criteria=u2 > Threshold  SaturateOnIntegerOverflow=off  InputSameDT=off
  Switch2 : Switch  Criteria=u2 > Threshold  SaturateOnIntegerOverflow=off  InputSameDT=off
  N_Sector : Outport
  wires:
  Uref1/1 -> Switch/2
  Uref2/1 -> Switch1/2
  Uref3/1 -> Switch2/2
  ConstanT1/1 -> Switch2/3, Switch/3, Switch1/3
  Constant/1 -> Switch2/1, Switch1/1, Switch/1
  Switch1/1 -> Gain1/1
  Switch/1 -> Gain/1
  Switch2/1 -> Gain2/1
  Add/1 -> N_Sector/1
  Gain/1 -> Add/1
  Gain1/1 -> Add/2
  Gain2/1 -> Add/3

== system PMSM_Simulation/Subsystem/Subsystem/SVM_PU/N_Sector_calc/Uref_Calc ==
  Ualpha : Inport
  Ubeta : Inport  Port=2
  Add : Sum  Inputs=+-
  Add1 : Sum  Inputs=--
  ConstanT1 : Constant  Value=sqrt(1)/2  OutDataTypeStr=single
  Constant : Constant  Value=sqrt(3)/2  OutDataTypeStr=single
  ProducT1 : Product
  Product : Product
  Signal Copy : SignalConversion  OverrideOpt=off
  Uref1 : Outport
  Uref2 : Outport  Port=2
  Uref3 : Outport  Port=3
  wires:
  Ubeta/1 -> ProducT1/1, Signal Copy/1
  Signal Copy/1 -> Uref1/1
  Ualpha/1 -> Product/1
  Constant/1 -> Product/2
  ConstanT1/1 -> ProducT1/2
  Product/1 -> Add1/1, Add/1
  ProducT1/1 -> Add1/2, Add/2
  Add/1 -> Uref2/1
  Add1/1 -> Uref3/1

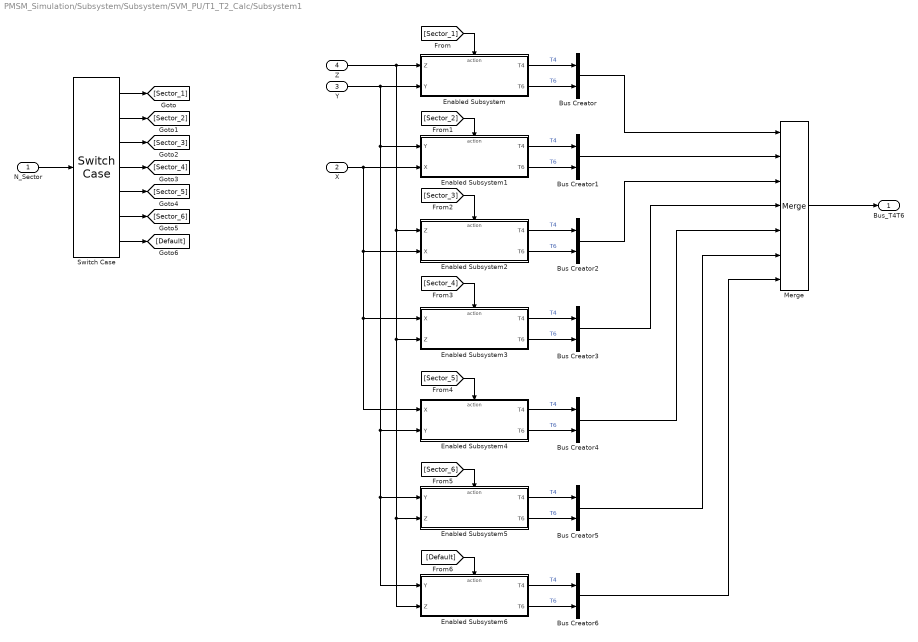
== system PMSM_Simulation/Subsystem/Subsystem/SVM_PU/T1_T2_Calc/Subsystem1 ==
  N_Sector : Inport
  X : Inport  Port=2
  Y : Inport  Port=3
  Z : Inport  Port=4
  Bus Creator{,1..6} (7 alike) : BusCreator  Inputs=2
  Enabled Subsystem : Subsystem  TreatAsAtomicUnit=on
  Enabled Subsystem1 : Subsystem  TreatAsAtomicUnit=on
  Enabled Subsystem2 : Subsystem  TreatAsAtomicUnit=on
  Enabled Subsystem3 : Subsystem  TreatAsAtomicUnit=on
  Enabled Subsystem4 : Subsystem  TreatAsAtomicUnit=on
  Enabled Subsystem5 : Subsystem  TreatAsAtomicUnit=on
  Enabled Subsystem6 : Subsystem  TreatAsAtomicUnit=on
  Merge : Merge  Inputs=7
  Switch Case : SwitchCase  CaseConditions={1,2,3,4,5,6}
  Bus_T4T6 : Outport
  wires:
  N_Sector/1 -> Switch Case/1
  Switch Case/1 -> [Sector_1]
  Switch Case/2 -> [Sector_2]
  Switch Case/3 -> [Sector_3]
  Switch Case/4 -> [Sector_4]
  Switch Case/5 -> [Sector_5]
  Switch Case/6 -> [Sector_6]
  Switch Case/7 -> [Default]
  [Sector_1] -> Enabled Subsystem/Action
  Y/1 -> Enabled Subsystem6/1(Y), Enabled Subsystem5/1(Y), Enabled Subsystem4/2(Y), Enabled Subsystem1/1(Y), Enabled Subsystem/2(Y)
  Z/1 -> Enabled Subsystem3/2(Z), Enabled Subsystem6/2(Z), Enabled Subsystem5/2(Z), Enabled Subsystem2/1(Z), Enabled Subsystem/1(Z)
  [Sector_2] -> Enabled Subsystem1/Action
  X/1 -> Enabled Subsystem4/1(X), Enabled Subsystem3/1(X), Enabled Subsystem2/2(X), Enabled Subsystem1/2(X)
  [Sector_3] -> Enabled Subsystem2/Action
  [Sector_4] -> Enabled Subsystem3/Action
  [Sector_5] -> Enabled Subsystem4/Action
  [Sector_6] -> Enabled Subsystem5/Action
  [Default] -> Enabled Subsystem6/Action
  Enabled Subsystem/1(T4) -> Bus Creator/1  "T4"
  Enabled Subsystem/2(T6) -> Bus Creator/2  "T6"
  Enabled Subsystem1/2(T6) -> Bus Creator1/2  "T6"
  Enabled Subsystem1/1(T4) -> Bus Creator1/1  "T4"
  Enabled Subsystem2/1(T4) -> Bus Creator2/1  "T4"
  Enabled Subsystem3/1(T4) -> Bus Creator3/1  "T4"
  Enabled Subsystem2/2(T6) -> Bus Creator2/2  "T6"
  Enabled Subsystem3/2(T6) -> Bus Creator3/2  "T6"
  Enabled Subsystem4/1(T4) -> Bus Creator4/1  "T4"
  Enabled Subsystem5/1(T4) -> Bus Creator5/1  "T4"
  Enabled Subsystem4/2(T6) -> Bus Creator4/2  "T6"
  Enabled Subsystem5/2(T6) -> Bus Creator5/2  "T6"
  Enabled Subsystem6/1(T4) -> Bus Creator6/1  "T4"
  Enabled Subsystem6/2(T6) -> Bus Creator6/2  "T6"
  Bus Creator/1 -> Merge/1
  Bus Creator1/1 -> Merge/2
  Bus Creator2/1 -> Merge/3
  Bus Creator3/1 -> Merge/4
  Bus Creator4/1 -> Merge/5
  Bus Creator5/1 -> Merge/6
  Bus Creator6/1 -> Merge/7
  Merge/1 -> Bus_T4T6/1

== system PMSM_Simulation/Subsystem/Subsystem/SVM_PU/T1_T2_Calc/Subsystem2 ==
  Bus_T4T6 : Inport
  Add : Sum
  Bus Selector : BusSelector  OutputSignals=T4,T6
  Bus_T4T1 : InportShadow
  Bus_T4T2 : InportShadow
  Bus_T4T3 : InportShadow
  If : If  IfExpression=u1 > 1.154  ElseIfExpressions=u1 > 1
  If Action Subsystem : Subsystem  TreatAsAtomicUnit=on
  If Action Subsystem1 : Subsystem  TreatAsAtomicUnit=on
  If Action Subsystem2 : Subsystem  TreatAsAtomicUnit=on
  Merge : Merge  Inputs=3
  Merge1 : Merge  Inputs=3
  T1 : Outport
  T2 : Outport  Port=2
  wires:
  Bus_T4T6/1 -> Bus Selector/1
  Bus Selector/1 -> Add/1  "<T4>"
  Bus Selector/2 -> Add/2  "<T6>"
  Add/1 -> If/1
  If/3 -> If Action Subsystem/Action
  If/2 -> If Action Subsystem1/Action
  If/1 -> If Action Subsystem2/Action
  Bus_T4T1/1 -> If Action Subsystem/1(Bus_T4T6)
  Bus_T4T2/1 -> If Action Subsystem1/1(Bus_T4T6)
  Bus_T4T3/1 -> If Action Subsystem2/1(Bus_T4T6)
  Merge/1 -> T1/1
  If Action Subsystem2/1(T1) -> Merge/1
  If Action Subsystem1/1(T1) -> Merge/2
  If Action Subsystem/1(T1) -> Merge/3
  If Action Subsystem2/2(T2) -> Merge1/1
  If Action Subsystem1/2(T2) -> Merge1/2
  If Action Subsystem/2(T2) -> Merge1/3
  Merge1/1 -> T2/1

== system PMSM_Simulation/Subsystem/Subsystem/SVM_PU/T1_T2_Calc/T4_T6 ==
  T4 : Inport
  T6 : Inport  Port=2
  Add : Sum
  Divide : Product  Inputs=*/
  Divide1 : Product  Inputs=*/
  Mux : Mux  Inputs=2
  Mux1 : Mux  Inputs=2
  Switch : Switch  Criteria=u2 > Threshold  Threshold=1  SaturateOnIntegerOverflow=off  InputSameDT=off
  T4_T6 : Outport
  wires:
  T4/1 -> Add/1, Mux1/1, Divide/1
  T6/1 -> Mux1/2, Add/2, Divide1/1
  Add/1 -> Divide1/2, Divide/2, Switch/2
  Divide/1 -> Mux/1  "T4"
  Divide1/1 -> Mux/2  "T6"
  Mux/1 -> Switch/1
  Mux1/1 -> Switch/3
  Switch/1 -> T4_T6/1

== system PMSM_Simulation/Subsystem/Subsystem/SVM_PU/Tcm_Calc/If Action Subsystem ==
  Ta : Inport
  Tb : Inport  Port=2
  Tc : Inport  Port=3
  Action Port : ActionPort  ActionPortLabel=case [ 1 ]:
  Tcm1 : Outport
  Tcm2 : Outport  Port=2
  Tcm3 : Outport  Port=3
  wires:
  Tb/1 -> Tcm1/1
  Ta/1 -> Tcm2/1
  Tc/1 -> Tcm3/1

== system PMSM_Simulation/Subsystem/Subsystem/SVM_PU/Tcm_Calc/If Action Subsystem1 ==
  Ta : Inport
  Tb : Inport  Port=2
  Tc : Inport  Port=3
  Action Port : ActionPort  ActionPortLabel=case [ 3 ]:
  Tcm1 : Outport
  Tcm2 : Outport  Port=2
  Tcm3 : Outport  Port=3
  wires:
  Ta/1 -> Tcm1/1
  Tb/1 -> Tcm2/1
  Tc/1 -> Tcm3/1

== system PMSM_Simulation/Subsystem/Subsystem/SVM_PU/Tcm_Calc/If Action Subsystem2 ==
  Ta : Inport
  Tb : Inport  Port=2
  Tc : Inport  Port=3
  Action Port : ActionPort  ActionPortLabel=case [ 4 ]:
  Tcm1 : Outport
  Tcm2 : Outport  Port=2
  Tcm3 : Outport  Port=3
  wires:
  Tc/1 -> Tcm1/1
  Tb/1 -> Tcm2/1
  Ta/1 -> Tcm3/1

== system PMSM_Simulation/Subsystem/Subsystem/SVM_PU/Tcm_Calc/If Action Subsystem3 ==
  Ta : Inport
  Tb : Inport  Port=2
  Tc : Inport  Port=3
  Action Port : ActionPort  ActionPortLabel=case [ 5 ]:
  Tcm1 : Outport
  Tcm2 : Outport  Port=2
  Tcm3 : Outport  Port=3
  wires:
  Tc/1 -> Tcm1/1
  Tb/1 -> Tcm3/1
  Ta/1 -> Tcm2/1

== system PMSM_Simulation/Subsystem/Subsystem/SVM_PU/Tcm_Calc/If Action Subsystem4 ==
  Ta : Inport
  Tb : Inport  Port=2
  Tc : Inport  Port=3
  Action Port : ActionPort  ActionPortLabel=case [ 6 ]:
  Tcm1 : Outport
  Tcm2 : Outport  Port=2
  Tcm3 : Outport  Port=3
  wires:
  Tc/1 -> Tcm2/1
  Tb/1 -> Tcm1/1
  Ta/1 -> Tcm3/1

== system PMSM_Simulation/Subsystem/Subsystem/SVM_PU/Tcm_Calc/If Action Subsystem5 ==
  Ta : Inport
  Tb : Inport  Port=2
  Tc : Inport  Port=3
  Action Port : ActionPort  ActionPortLabel=default:
  Tcm1 : Outport
  Tcm2 : Outport  Port=2
  Tcm3 : Outport  Port=3
  wires:
  Tc/1 -> Tcm2/1
  Tb/1 -> Tcm1/1
  Ta/1 -> Tcm3/1

== system PMSM_Simulation/Subsystem/Subsystem/SVM_PU/Tcm_Calc/If Action Subsystem7 ==
  Ta : Inport
  Tb : Inport  Port=2
  Tc : Inport  Port=3
  Action Port : ActionPort  ActionPortLabel=case [ 2 ]:
  Tcm1 : Outport
  Tcm2 : Outport  Port=2
  Tcm3 : Outport  Port=3
  wires:
  Ta/1 -> Tcm1/1
  Tc/1 -> Tcm2/1
  Tb/1 -> Tcm3/1

== system PMSM_Simulation/Subsystem/Subsystem/Subsystem2/Subsystem/DeadTimeDuty_Calc ==
  PwmFreq_Hz : Inport
  Constant : Constant  Value=KfDeadCompen_SetDeltaTime_us  OutDataTypeStr=single
  Constant1 : Constant  Value=1e6  OutDataTypeStr=single
  Divide2 : Product  Inputs=**/
  DeadTimeDuty_NULL : Outport
  wires:
  Divide2/1 -> DeadTimeDuty_NULL/1  "DeadTimeDuty_NULL"
  Constant/1 -> Divide2/1
  Constant1/1 -> Divide2/3
  PwmFreq_Hz/1 -> Divide2/2

== system PMSM_Simulation/Subsystem/Subsystem/Subsystem2/Subsystem/DeltaTimeOnOffDuty_Calc ==
  iPhase_U : Inport
  iPhase_V : Inport  Port=2
  iPhase_W : Inport  Port=3
  PwmFreq_Hz : Inport  Port=4
  1-D Lookup Table : Lookup_n-D  Priority=40  NumberOfTableDimensions=1  BreakpointsForDimension1="[0.0\t10.0\t20.0\t50.0\t100.0\t200.0\t400.0\t600.0]"  Table=single([0 0 0 0 0 0 0 0])  InternalRulePriority=Speed  RndMeth=Simplest
  1-D Lookup Table1 : Lookup_n-D  Priority=48  Commented=on  NumberOfTableDimensions=1  BreakpointsForDimension1="[0.0\t10.0\t20.0\t50.0\t100.0\t200.0\t400.0\t600.0]"  Table=single([1.9 1.6 1.25 0.9 0.82 0.67 0.61 0.54])  InternalRulePriority=Speed  RndMeth=Simplest
  1-D Lookup Table2 : Lookup_n-D  Priority=40  NumberOfTableDimensions=1  BreakpointsForDimension1="[0.0\t10.0\t20.0\t50.0\t100.0\t200.0\t400.0\t600.0]"  Table=single([0 0 0 0 0 0 0 0])  InternalRulePriority=Speed  RndMeth=Simplest
  1-D Lookup Table3 : Lookup_n-D  Priority=40  NumberOfTableDimensions=1  BreakpointsForDimension1="[0.0\t10.0\t20.0\t50.0\t100.0\t200.0\t400.0\t600.0]"  Table=single([0 0 0 0 0 0 0 0])  InternalRulePriority=Speed  RndMeth=Simplest
  Abs : Abs  Priority=39  SaturateOnIntegerOverflow=off
  Abs1 : Abs  Priority=47  SaturateOnIntegerOverflow=off
  Abs2 : Abs  Priority=51  SaturateOnIntegerOverflow=off
  Bus Creator : BusCreator  Inputs=3
  Constant : Constant  Value=1e6  OutDataTypeStr=single
  Divide : Product  Inputs=**/
  Divide1 : Product  Inputs=**/
  Divide2 : Product  Inputs=**/
  Bus_DeltaTimeOnOffDuty : Outport
  wires:
  1-D Lookup Table/1 -> Divide/1
  1-D Lookup Table3/1 -> Divide2/1
  PwmFreq_Hz/1 -> Divide/2, Divide1/2, Divide2/2
  iPhase_U/1 -> Abs/1
  1-D Lookup Table2/1 -> Divide1/1
  Bus Creator/1 -> Bus_DeltaTimeOnOffDuty/1
  Abs2/1 -> 1-D Lookup Table3/1  "iPhaseAbs"
  iPhase_V/1 -> Abs1/1
  Constant/1 -> Divide/3, Divide1/3, Divide2/3
  Abs1/1 -> 1-D Lookup Table2/1  "iPhaseAbs"
  Abs/1 -> 1-D Lookup Table/1  "iPhaseAbs"
  Divide1/1 -> Bus Creator/2  "DeltaTimeOnOffV_NULL"
  Divide/1 -> Bus Creator/1  "DeltaTimeOnOffU_NULL"
  Divide2/1 -> Bus Creator/3  "DeltaTimeOnOffW_NULL"
  iPhase_W/1 -> Abs2/1

== system PMSM_Simulation/Subsystem/Subsystem/Subsystem2/Subsystem/DutyErr_Calc ==
  Bus_DutyAvon : Inport
  Bus_DeltaTimeOnOffDuty : Inport  Port=2
  DeadTimeDuty : Inport  Port=3
  Bus Creator : BusCreator  Inputs=3
  PhaseU : Subsystem
  PhaseV : Subsystem
  PhaseW : Subsystem
  Bus_DutyCompensate : Outport
  wires:
  Bus_DutyAvon/1 -> PhaseW/1(Bus_DutyAvon), PhaseV/1(Bus_DutyAvon), PhaseU/1(Bus_DutyAvon)
  Bus_DeltaTimeOnOffDuty/1 -> PhaseW/2(Bus_DeltaTimeOnOffDuty), PhaseV/2(Bus_DeltaTimeOnOffDuty), PhaseU/2(Bus_DeltaTimeOnOffDuty)
  DeadTimeDuty/1 -> PhaseW/3(DeadTimeDuty), PhaseV/3(DeadTimeDuty), PhaseU/3(DeadTimeDuty)
  PhaseV/1(DutyCompensate_V) -> Bus Creator/2  "DutyCompensate_V"
  PhaseU/1(DutyCompensate_U) -> Bus Creator/1  "DutyCompensate_U"
  PhaseW/1(DutyCompensate_W) -> Bus Creator/3  "DutyCompensate_W"
  Bus Creator/1 -> Bus_DutyCompensate/1

== system PMSM_Simulation/Subsystem/Subsystem/Subsystem2/Subsystem/Tavon_Calc ==
  U_Phase_Dyc : Inport
  V_Phase_Dyc : Inport  Port=2
  W_Phase_Dyc : Inport  Port=3
  iPhase_U : Inport  Port=4
  iPhase_V : Inport  Port=5
  iPhase_W : Inport  Port=6
  uDcLink : Inport  Port=7
  Bus Creator : BusCreator  Inputs=3
  ia : Subsystem
  ia1 : Subsystem
  ia2 : Subsystem
  Bus_DutyAvon : Outport
  wires:
  V_Phase_Dyc/1 -> ia1/2(Phase_Dyc)
  ia1/1("Duty_Avon ") -> Bus Creator/2  "DutyAvon_V"
  U_Phase_Dyc/1 -> ia/2(Phase_Dyc)
  uDcLink/1 -> ia2/3(uDcLink), ia1/3(uDcLink), ia/3(uDcLink)
  iPhase_V/1 -> ia1/1(iPhase)
  ia2/1("Duty_Avon ") -> Bus Creator/3  "DutyAvon_W"
  iPhase_W/1 -> ia2/1(iPhase)
  W_Phase_Dyc/1 -> ia2/2(Phase_Dyc)
  Bus Creator/1 -> Bus_DutyAvon/1  "DutyAvon"
  iPhase_U/1 -> ia/1(iPhase)
  ia/1("Duty_Avon ") -> Bus Creator/1  "DutyAvon_U"

== system PMSM_Simulation/Subsystem/Subsystem/Subsystem2/Subsystem1/Switch Case Action Subsystem ==
  Bus_DutyCompensate : Inport
  Action Port : ActionPort  ActionPortLabel=case [ 0 ]:
  Add : Sum  Inputs=++-
  Add1 : Sum  Inputs=+-+
  Add2 : Sum  Inputs=+-+
  Bus Creator : BusCreator  Inputs=3
  Bus Selector : BusSelector  OutputSignals=Bus_DutyAvon.DutyAvon_U,DeadTimeDuty_NULL,Bus_DeltaTimeOnOffDuty.DeltaTimeOnOffU_NULL
  Bus Selector1 : BusSelector  OutputSignals=Bus_DutyAvon.DutyAvon_V,DeadTimeDuty_NULL,Bus_DeltaTimeOnOffDuty.DeltaTimeOnOffV_NULL
  Bus Selector2 : BusSelector  OutputSignals=Bus_DutyAvon.DutyAvon_W,DeadTimeDuty_NULL,Bus_DeltaTimeOnOffDuty.DeltaTimeOnOffW_NULL
  PwmDuty : Outport
  wires:
  Add/1 -> Bus Creator/1  "uDuty"
  Add1/1 -> Bus Creator/2  "vDuty"
  Add2/1 -> Bus Creator/3  "wDuty"
  Bus Creator/1 -> PwmDuty/1
  Bus_DutyCompensate/1 -> Bus Selector/1, Bus Selector2/1, Bus Selector1/1
  Bus Selector/1 -> Add/1  "<DutyAvon_U>"
  Bus Selector/3 -> Add/3  "<DeltaTimeOnOffU_NULL>"
  Bus Selector1/2 -> Add1/2  "<DeadTimeDuty_NULL>"
  Bus Selector1/1 -> Add1/1  "<DutyAvon_V>"
  Bus Selector2/1 -> Add2/1  "<DutyAvon_W>"
  Bus Selector2/2 -> Add2/2  "<DeadTimeDuty_NULL>"
  Bus Selector/2 -> Add/2  "<DeadTimeDuty_NULL>"
  Bus Selector1/3 -> Add1/3  "<DeltaTimeOnOffV_NULL>"
  Bus Selector2/3 -> Add2/3  "<DeltaTimeOnOffW_NULL>"

== system PMSM_Simulation/Subsystem/Subsystem/Subsystem2/Subsystem1/Switch Case Action Subsystem1 ==
  Bus_DutyCompensate : Inport
  Action Port : ActionPort  ActionPortLabel=case [ 1 ]:
  Add : Sum  Inputs=++-
  Add1 : Sum  Inputs=++-
  Add2 : Sum  Inputs=+-+
  Bus Creator : BusCreator  Inputs=3
  Bus Selector : BusSelector  OutputSignals=Bus_DutyAvon.DutyAvon_U,DeadTimeDuty_NULL,Bus_DeltaTimeOnOffDuty.DeltaTimeOnOffU_NULL
  Bus Selector1 : BusSelector  OutputSignals=Bus_DutyAvon.DutyAvon_V,DeadTimeDuty_NULL,Bus_DeltaTimeOnOffDuty.DeltaTimeOnOffV_NULL
  Bus Selector2 : BusSelector  OutputSignals=Bus_DutyAvon.DutyAvon_W,DeadTimeDuty_NULL,Bus_DeltaTimeOnOffDuty.DeltaTimeOnOffW_NULL
  PwmDuty : Outport
  wires:
  Add/1 -> Bus Creator/1  "uDuty"
  Add1/1 -> Bus Creator/2  "vDuty"
  Add2/1 -> Bus Creator/3  "wDuty"
  Bus Creator/1 -> PwmDuty/1
  Bus_DutyCompensate/1 -> Bus Selector/1, Bus Selector2/1, Bus Selector1/1
  Bus Selector/1 -> Add/1  "<DutyAvon_U>"
  Bus Selector/3 -> Add/3  "<DeltaTimeOnOffU_NULL>"
  Bus Selector1/2 -> Add1/2  "<DeadTimeDuty_NULL>"
  Bus Selector1/1 -> Add1/1  "<DutyAvon_V>"
  Bus Selector2/1 -> Add2/1  "<DutyAvon_W>"
  Bus Selector2/2 -> Add2/2  "<DeadTimeDuty_NULL>"
  Bus Selector/2 -> Add/2  "<DeadTimeDuty_NULL>"
  Bus Selector1/3 -> Add1/3  "<DeltaTimeOnOffV_NULL>"
  Bus Selector2/3 -> Add2/3  "<DeltaTimeOnOffW_NULL>"

== system PMSM_Simulation/Subsystem/Subsystem/Subsystem2/Subsystem1/Switch Case Action Subsystem2 ==
  Bus_DutyCompensate : Inport
  Action Port : ActionPort  ActionPortLabel=case [ 2 ]:
  Add : Sum  Inputs=+-+
  Add1 : Sum  Inputs=++-
  Add2 : Sum  Inputs=+-+
  Bus Creator : BusCreator  Inputs=3
  Bus Selector : BusSelector  OutputSignals=Bus_DutyAvon.DutyAvon_U,DeadTimeDuty_NULL,Bus_DeltaTimeOnOffDuty.DeltaTimeOnOffU_NULL
  Bus Selector1 : BusSelector  OutputSignals=Bus_DutyAvon.DutyAvon_V,DeadTimeDuty_NULL,Bus_DeltaTimeOnOffDuty.DeltaTimeOnOffV_NULL
  Bus Selector2 : BusSelector  OutputSignals=Bus_DutyAvon.DutyAvon_W,DeadTimeDuty_NULL,Bus_DeltaTimeOnOffDuty.DeltaTimeOnOffW_NULL
  PwmDuty : Outport
  wires:
  Add/1 -> Bus Creator/1  "uDuty"
  Add1/1 -> Bus Creator/2  "vDuty"
  Add2/1 -> Bus Creator/3  "wDuty"
  Bus Creator/1 -> PwmDuty/1
  Bus_DutyCompensate/1 -> Bus Selector/1, Bus Selector2/1, Bus Selector1/1
  Bus Selector/1 -> Add/1  "<DutyAvon_U>"
  Bus Selector/3 -> Add/3  "<DeltaTimeOnOffU_NULL>"
  Bus Selector1/2 -> Add1/2  "<DeadTimeDuty_NULL>"
  Bus Selector1/1 -> Add1/1  "<DutyAvon_V>"
  Bus Selector2/1 -> Add2/1  "<DutyAvon_W>"
  Bus Selector2/2 -> Add2/2  "<DeadTimeDuty_NULL>"
  Bus Selector/2 -> Add/2  "<DeadTimeDuty_NULL>"
  Bus Selector1/3 -> Add1/3  "<DeltaTimeOnOffV_NULL>"
  Bus Selector2/3 -> Add2/3  "<DeltaTimeOnOffW_NULL>"

== system PMSM_Simulation/Subsystem/Subsystem/Subsystem2/Subsystem1/Switch Case Action Subsystem3 ==
  Bus_DutyCompensate : Inport
  Action Port : ActionPort  ActionPortLabel=case [ 3 ]:
  Add : Sum  Inputs=+-+
  Add1 : Sum  Inputs=++-
  Add2 : Sum  Inputs=++-
  Bus Creator : BusCreator  Inputs=3
  Bus Selector : BusSelector  OutputSignals=Bus_DutyAvon.DutyAvon_U,DeadTimeDuty_NULL,Bus_DeltaTimeOnOffDuty.DeltaTimeOnOffU_NULL
  Bus Selector1 : BusSelector  OutputSignals=Bus_DutyAvon.DutyAvon_V,DeadTimeDuty_NULL,Bus_DeltaTimeOnOffDuty.DeltaTimeOnOffV_NULL
  Bus Selector2 : BusSelector  OutputSignals=Bus_DutyAvon.DutyAvon_W,DeadTimeDuty_NULL,Bus_DeltaTimeOnOffDuty.DeltaTimeOnOffW_NULL
  PwmDuty : Outport
  wires:
  Add/1 -> Bus Creator/1  "uDuty"
  Add1/1 -> Bus Creator/2  "vDuty"
  Add2/1 -> Bus Creator/3  "wDuty"
  Bus Creator/1 -> PwmDuty/1
  Bus_DutyCompensate/1 -> Bus Selector/1, Bus Selector2/1, Bus Selector1/1
  Bus Selector/1 -> Add/1  "<DutyAvon_U>"
  Bus Selector/3 -> Add/3  "<DeltaTimeOnOffU_NULL>"
  Bus Selector1/2 -> Add1/2  "<DeadTimeDuty_NULL>"
  Bus Selector1/1 -> Add1/1  "<DutyAvon_V>"
  Bus Selector2/1 -> Add2/1  "<DutyAvon_W>"
  Bus Selector2/2 -> Add2/2  "<DeadTimeDuty_NULL>"
  Bus Selector/2 -> Add/2  "<DeadTimeDuty_NULL>"
  Bus Selector1/3 -> Add1/3  "<DeltaTimeOnOffV_NULL>"
  Bus Selector2/3 -> Add2/3  "<DeltaTimeOnOffW_NULL>"

== system PMSM_Simulation/Subsystem/Subsystem/Subsystem2/Subsystem1/Switch Case Action Subsystem4 ==
  Bus_DutyCompensate : Inport
  Action Port : ActionPort  ActionPortLabel=case [ 4 ]:
  Add : Sum  Inputs=+-+
  Add1 : Sum  Inputs=+-+
  Add2 : Sum  Inputs=++-
  Bus Creator : BusCreator  Inputs=3
  Bus Selector : BusSelector  OutputSignals=Bus_DutyAvon.DutyAvon_U,DeadTimeDuty_NULL,Bus_DeltaTimeOnOffDuty.DeltaTimeOnOffU_NULL
  Bus Selector1 : BusSelector  OutputSignals=Bus_DutyAvon.DutyAvon_V,DeadTimeDuty_NULL,Bus_DeltaTimeOnOffDuty.DeltaTimeOnOffV_NULL
  Bus Selector2 : BusSelector  OutputSignals=Bus_DutyAvon.DutyAvon_W,DeadTimeDuty_NULL,Bus_DeltaTimeOnOffDuty.DeltaTimeOnOffW_NULL
  PwmDuty : Outport
  wires:
  Add/1 -> Bus Creator/1  "uDuty"
  Add1/1 -> Bus Creator/2  "vDuty"
  Add2/1 -> Bus Creator/3  "wDuty"
  Bus Creator/1 -> PwmDuty/1
  Bus_DutyCompensate/1 -> Bus Selector/1, Bus Selector2/1, Bus Selector1/1
  Bus Selector/1 -> Add/1  "<DutyAvon_U>"
  Bus Selector/3 -> Add/3  "<DeltaTimeOnOffU_NULL>"
  Bus Selector1/2 -> Add1/2  "<DeadTimeDuty_NULL>"
  Bus Selector1/1 -> Add1/1  "<DutyAvon_V>"
  Bus Selector2/1 -> Add2/1  "<DutyAvon_W>"
  Bus Selector2/2 -> Add2/2  "<DeadTimeDuty_NULL>"
  Bus Selector/2 -> Add/2  "<DeadTimeDuty_NULL>"
  Bus Selector1/3 -> Add1/3  "<DeltaTimeOnOffV_NULL>"
  Bus Selector2/3 -> Add2/3  "<DeltaTimeOnOffW_NULL>"

== system PMSM_Simulation/Subsystem/Subsystem/Subsystem2/Subsystem1/Switch Case Action Subsystem5 ==
  Bus_DutyCompensate : Inport
  Action Port : ActionPort  ActionPortLabel=case [ 5 ]:
  Add : Sum  Inputs=++-
  Add1 : Sum  Inputs=+-+
  Add2 : Sum  Inputs=++-
  Bus Creator : BusCreator  Inputs=3
  Bus Selector : BusSelector  OutputSignals=Bus_DutyAvon.DutyAvon_U,DeadTimeDuty_NULL,Bus_DeltaTimeOnOffDuty.DeltaTimeOnOffU_NULL
  Bus Selector1 : BusSelector  OutputSignals=Bus_DutyAvon.DutyAvon_V,DeadTimeDuty_NULL,Bus_DeltaTimeOnOffDuty.DeltaTimeOnOffV_NULL
  Bus Selector2 : BusSelector  OutputSignals=Bus_DutyAvon.DutyAvon_W,DeadTimeDuty_NULL,Bus_DeltaTimeOnOffDuty.DeltaTimeOnOffW_NULL
  PwmDuty : Outport
  wires:
  Add/1 -> Bus Creator/1  "uDuty"
  Add1/1 -> Bus Creator/2  "vDuty"
  Add2/1 -> Bus Creator/3  "wDuty"
  Bus Creator/1 -> PwmDuty/1
  Bus_DutyCompensate/1 -> Bus Selector/1, Bus Selector2/1, Bus Selector1/1
  Bus Selector/1 -> Add/1  "<DutyAvon_U>"
  Bus Selector/3 -> Add/3  "<DeltaTimeOnOffU_NULL>"
  Bus Selector1/2 -> Add1/2  "<DeadTimeDuty_NULL>"
  Bus Selector1/1 -> Add1/1  "<DutyAvon_V>"
  Bus Selector2/1 -> Add2/1  "<DutyAvon_W>"
  Bus Selector2/2 -> Add2/2  "<DeadTimeDuty_NULL>"
  Bus Selector/2 -> Add/2  "<DeadTimeDuty_NULL>"
  Bus Selector1/3 -> Add1/3  "<DeltaTimeOnOffV_NULL>"
  Bus Selector2/3 -> Add2/3  "<DeltaTimeOnOffW_NULL>"

== system PMSM_Simulation/Subsystem/Subsystem/Subsystem2/Subsystem1/Switch Case Action Subsystem8 ==
  "Bus_DutyCorr " : Inport
  Action Port : ActionPort  ActionPortLabel=default:
  Bus Creator : BusCreator  Inputs=3
  Bus Selector : BusSelector  OutputSignals=SVM_DutyPhase.DutyPhaseU,SVM_DutyPhase.DutyPhaseV,SVM_DutyPhase.DutyPhaseW
  Signal Copy : SignalConversion  OverrideOpt=off
  Signal Copy1 : SignalConversion  OverrideOpt=off
  Signal Copy2 : SignalConversion  OverrideOpt=off
  PwmDuty : Outport
  wires:
  "Bus_DutyCorr "/1 -> Bus Selector/1
  Bus Selector/1 -> Signal Copy/1  "<DutyPhaseU>"
  Signal Copy1/1 -> Bus Creator/2  "vDuty"
  Bus Creator/1 -> PwmDuty/1
  Signal Copy2/1 -> Bus Creator/3  "wDuty"
  Signal Copy/1 -> Bus Creator/1  "uDuty"
  Bus Selector/2 -> Signal Copy1/1  "<DutyPhaseV>"
  Bus Selector/3 -> Signal Copy2/1  "<DutyPhaseW>"

== system PMSM_Simulation/Subsystem/Subsystem/Subsystem2/Subsystem2/Subsystem1 ==
  IsdDes_A : Inport
  IsqDes_A : Inport  Port=2
  IsdFb_A : Inport  Port=3
  IsqFb_A : Inport  Port=4
  Bus Creator : BusCreator  Inputs=2
  Bus Creator1 : BusCreator  Inputs=2
  Bus Selector : BusSelector  OutputSignals=Isd_A,Isq_A
  Constant : Constant  Value=VbDeadComp_SwtUseIsttrDes_flg
  Switch : Switch  Criteria=u2 ~= 0  SaturateOnIntegerOverflow=off  InputSameDT=off
  Isd_A : Outport
  Isq_A : Outport  Port=2
  wires:
  Bus Creator1/1 -> Switch/3
  IsqDes_A/1 -> Bus Creator/2  "Isq_A"
  Bus Creator/1 -> Switch/1
  IsqFb_A/1 -> Bus Creator1/2  "Isq_A"
  IsdFb_A/1 -> Bus Creator1/1  "Isd_A"
  Constant/1 -> Switch/2
  IsdDes_A/1 -> Bus Creator/1  "Isd_A"
  Switch/1 -> Bus Selector/1
  Bus Selector/1 -> Isd_A/1  "<Isd_A>"
  Bus Selector/2 -> Isq_A/1  "<Isq_A>"
